simulink model "Ejemplo0421_Controlador_a"  (R2025b)
settings: Solver=VariableStepAuto  StartTime=0.0  StopTime=30  RelTol=1e-3
settings Model: Creator=cjuar  LastModifiedBy=cjuar

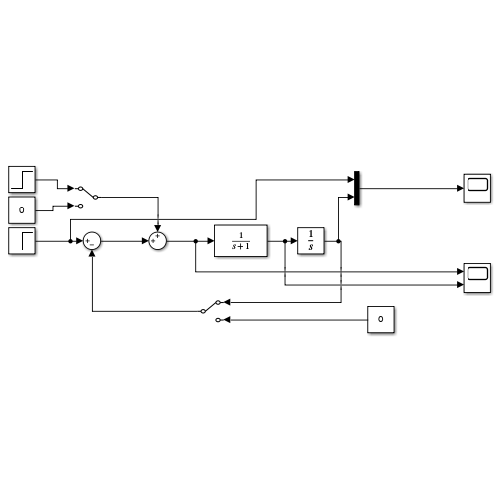
[thumbnail: Simulink's stored preview of the top-level diagram]
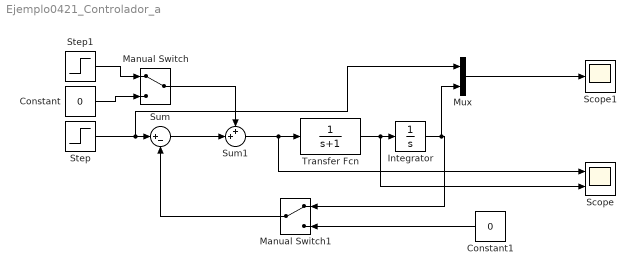
== system Ejemplo0421_Controlador_a ==
  Constant : Constant  Value=0
  Constant1 : Constant  Value=0
  Integrator : Integrator
  Manual Switch : ManualSwitch
  Manual Switch1 : ManualSwitch
  Mux : Mux  Inputs=2
  Scope : Scope  NumInputPorts=2
      settings: ActiveDisplayYMinimum=-0.30853115503001827  ActiveDisplayYMaximum=1.146057773924223
  Scope1 : Scope
      settings: ActiveDisplayYMinimum=-0.27038403276682421  ActiveDisplayYMaximum=2.4334562949014185
  Step : Step  SampleTime=0
  Step1 : Step  Time=15  SampleTime=0
  Sum : Sum  Inputs=|+-
  Sum1 : Sum  Inputs=++|
  Transfer Fcn : TransferFcn  Denominator=[1 1]
  wires:
  Transfer Fcn/1 -> Scope/2, Integrator/1
  Integrator/1 -> Mux/2, Manual Switch1/1
  Sum1/1 -> Scope/1, Transfer Fcn/1
  Step/1 -> Mux/1, Sum/1
  Sum/1 -> Sum1/2
  Manual Switch/1 -> Sum1/1
  Step1/1 -> Manual Switch/1
  Constant/1 -> Manual Switch/2
  Manual Switch1/1 -> Sum/2
  Constant1/1 -> Manual Switch1/2
  Mux/1 -> Scope1/1
